simulink model "proba1"  (Simulink 7.0)
settings: Solver=ode1  StartTime=0.0  StopTime=Inf  FixedStep=0.001  RelTol=1e-3
PostLoadFcn:
  | ,try, rti_mdl_postloadfcn(bdroot, 'UpdateModel', 280, 'rti1005'); catch, disp(lasterr); end,
libraries: simulink x27, simulink_extras x12, rtilibm x10
(part 1 of 2)
settings Model: Creator=k12_p800a  LastModifiedBy=k12_p800a  BufferReuse=off
settings OptimizationCC: BlockReduction=off  BooleanDataType=off  OptimizeBlockIOStorage=off  BufferReuse=off  ExpressionFolding=off  LocalBlockOutputs=off
settings HardwareCC: ProdIntDivRoundTo=Zero  ProdEndianess=BigEndian  ProdHWDeviceType=Specified  TargetIntDivRoundTo=Zero  TargetEndianess=BigEndian
settings RTWCC: SystemTargetFile=rti1005.tlc  MakeCommand=make_rti  TemplateMakefile=rti1005.tmf  Description=dSPACE DS1005 Hardware Platform  ProcessScript=rti1005_make_rtw_hook
settings STFCustomTargetCC: GenFloatMathFcnCalls=ANSI_C  ModelReferenceCompliant=off  SystemTargetFile=rti1005.tlc
settings GRTTargetCC: ModelReferenceCompliant=off  CompOptLevelCompliant=off  MatFileLogging=off  ExtModeMexFile=rti_comm_2
settings CustomProperty: DataType=RTWOptions_EnumType_C__dSPACE_60_matlab_rti1005_tlc_rti1005_InitialSimState  Value=RUN
settings EnumStrPairs: String=RUN

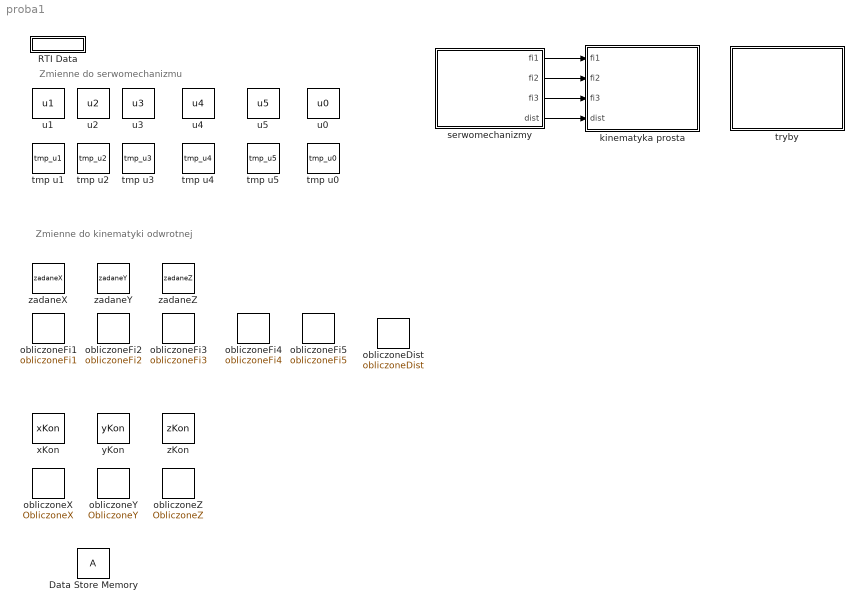
== system proba1 ==
  note: Zmienne do kinematyki odwrotnej
  note: Zmienne do serwomechanizmu
  Data Store Memory : DataStoreMemory  DataStoreName=A  ReadBeforeWriteMsg=warning  WriteAfterWriteMsg=warning  WriteAfterReadMsg=warning  OutDataType=sfix(16)  OutScaling=2^0
  RTI Data : Subsystem  Tag=struct('RTIDataServer',struct('RTIDataServerVs','2','RTIModelDescription','struct(''main'',''proba1'',''sub'','''',''isMp'',0)'))  LoadFcn="if exist('rtidc'), try,  rtidc('DataHostBlockClbLoad', gcbh); catch, disp(['Warning: ''LoadFcn'' for RTI Data block failed: ' lasterr]); end, end,"
      settings: CopyFcn="if exist('rtidc'), try,  rtidc('DataHostBlockClbCopy', gcbh); catch, disp(['Warning: ''CopyFcn'' for RTI Data block failed: ' lasterr]); end, end,"  DeleteFcn="if exist('rtidc'), try,  rtidc('DataHostBlockClbDelete', gcbh); catch, disp(['Warning: ''DeleteFcn'' for RTI Data block failed: ' lasterr]); end, end,"  ModelCloseFcn="if exist('rtidc'), try,  rtidc('DataHostBlockClbModelClose', gcbh); catch, disp(['Warning: ''ModelCloseFcn'' for RTI Data block failed: ' lasterr]); end, end,"  PreSaveFcn="if exist('rtidc'), try,  rtidc('DataHostBlockClbPreSave', gcbh); catch, disp(['Warning: ''PreSaveFcn'' for RTI Data block failed: ' lasterr]); end, end,"  PostSaveFcn="if exist('rtidc'), try,  rtidc('DataHostBlockClbPostSave', gcbh); catch, disp(['Warning: ''PostSaveFcn'' for RTI Data block failed: ' lasterr]); end, end,"  NameChangeFcn="if exist('rtidc'), try,  rtidc('DataHostBlockClbNameChange', gcbh); catch, disp(['Warning: ''NameChangeFcn'' for RTI Data block failed: ' lasterr]); end, end,"
      mask Type: RTI_DATA_HOST
      mask Description:
      | RTI Data Block.
      | This block is used by RTI to store internal model-dependent data.
      | Please keep this block on the root level of the model. Deleting this block will result in data loss.
      | 
      | NEVER DELETE OR COPY THIS BLOCK!
      mask Help:
      | RTI Data Block.
      | This block is used by RTI to store internal model-dependent data.
      | Please keep this block on the root level of the model. Deleting this block will result in data loss.
      | 
      | NEVER DELETE OR COPY THIS BLOCK!
      mask Display:
      | text(0.5, 0.5, 'RTI Data', 'HorizontalAlignment', 'center');
      | plot([1 0]);
  kinematyka prosta : Subsystem
  obliczoneDist : DataStoreMemory  DataStoreName=obliczoneDist  ReadBeforeWriteMsg=warning  WriteAfterWriteMsg=warning  WriteAfterReadMsg=warning
  obliczoneFi1 : DataStoreMemory  DataStoreName=obliczoneFi1  ReadBeforeWriteMsg=warning  WriteAfterWriteMsg=warning  WriteAfterReadMsg=warning
  obliczoneFi2 : DataStoreMemory  DataStoreName=obliczoneFi2  ReadBeforeWriteMsg=warning  WriteAfterWriteMsg=warning  WriteAfterReadMsg=warning
  obliczoneFi3 : DataStoreMemory  DataStoreName=obliczoneFi3  ReadBeforeWriteMsg=warning  WriteAfterWriteMsg=warning  WriteAfterReadMsg=warning
  obliczoneFi4 : DataStoreMemory  DataStoreName=obliczoneFi4  ReadBeforeWriteMsg=warning  WriteAfterWriteMsg=warning  WriteAfterReadMsg=warning
  obliczoneFi5 : DataStoreMemory  DataStoreName=obliczoneFi5  ReadBeforeWriteMsg=warning  WriteAfterWriteMsg=warning  WriteAfterReadMsg=warning
  obliczoneX : DataStoreMemory  DataStoreName=ObliczoneX  ReadBeforeWriteMsg=warning  WriteAfterWriteMsg=warning  WriteAfterReadMsg=warning
  obliczoneY : DataStoreMemory  DataStoreName=ObliczoneY  ReadBeforeWriteMsg=warning  WriteAfterWriteMsg=warning  WriteAfterReadMsg=warning
  obliczoneZ : DataStoreMemory  DataStoreName=ObliczoneZ  ReadBeforeWriteMsg=warning  WriteAfterWriteMsg=warning  WriteAfterReadMsg=warning
  serwomechanizmy : Subsystem
  tmp u0 : DataStoreMemory  DataStoreName=tmp_u0  ReadBeforeWriteMsg=warning  WriteAfterWriteMsg=warning  WriteAfterReadMsg=warning
  tmp u1 : DataStoreMemory  DataStoreName=tmp_u1  ReadBeforeWriteMsg=warning  WriteAfterWriteMsg=warning  WriteAfterReadMsg=warning
  tmp u2 : DataStoreMemory  DataStoreName=tmp_u2  ReadBeforeWriteMsg=warning  WriteAfterWriteMsg=warning  WriteAfterReadMsg=warning
  tmp u3 : DataStoreMemory  DataStoreName=tmp_u3  ReadBeforeWriteMsg=warning  WriteAfterWriteMsg=warning  WriteAfterReadMsg=warning
  tmp u4 : DataStoreMemory  DataStoreName=tmp_u4  ReadBeforeWriteMsg=warning  WriteAfterWriteMsg=warning  WriteAfterReadMsg=warning
  tmp u5 : DataStoreMemory  DataStoreName=tmp_u5  ReadBeforeWriteMsg=warning  WriteAfterWriteMsg=warning  WriteAfterReadMsg=warning
  tryby : Subsystem
  u0 : DataStoreMemory  DataStoreName=u0  ReadBeforeWriteMsg=warning  WriteAfterWriteMsg=warning  WriteAfterReadMsg=warning
  u1 : DataStoreMemory  DataStoreName=u1  ReadBeforeWriteMsg=warning  WriteAfterWriteMsg=warning  WriteAfterReadMsg=warning
  u2 : DataStoreMemory  DataStoreName=u2  ReadBeforeWriteMsg=warning  WriteAfterWriteMsg=warning  WriteAfterReadMsg=warning
  u3 : DataStoreMemory  DataStoreName=u3  ReadBeforeWriteMsg=warning  WriteAfterWriteMsg=warning  WriteAfterReadMsg=warning
  u4 : DataStoreMemory  DataStoreName=u4  ReadBeforeWriteMsg=warning  WriteAfterWriteMsg=warning  WriteAfterReadMsg=warning
  u5 : DataStoreMemory  DataStoreName=u5  ReadBeforeWriteMsg=warning  WriteAfterWriteMsg=warning  WriteAfterReadMsg=warning
  xKon : DataStoreMemory  DataStoreName=xKon  ReadBeforeWriteMsg=warning  WriteAfterWriteMsg=warning  WriteAfterReadMsg=warning
  yKon : DataStoreMemory  DataStoreName=yKon  ReadBeforeWriteMsg=warning  WriteAfterWriteMsg=warning  WriteAfterReadMsg=warning
  zKon : DataStoreMemory  DataStoreName=zKon  ReadBeforeWriteMsg=warning  WriteAfterWriteMsg=warning  WriteAfterReadMsg=warning
  zadaneX : DataStoreMemory  DataStoreName=zadaneX  ReadBeforeWriteMsg=warning  WriteAfterWriteMsg=warning  WriteAfterReadMsg=warning
  zadaneY : DataStoreMemory  DataStoreName=zadaneY  ReadBeforeWriteMsg=warning  WriteAfterWriteMsg=warning  WriteAfterReadMsg=warning
  zadaneZ : DataStoreMemory  DataStoreName=zadaneZ  ReadBeforeWriteMsg=warning  WriteAfterWriteMsg=warning  WriteAfterReadMsg=warning
  wires:
  serwomechanizmy/1(fi1) -> kinematyka prosta/1(fi1)
  serwomechanizmy/2(fi2) -> kinematyka prosta/2(fi2)
  serwomechanizmy/3(fi3) -> kinematyka prosta/3(fi3)
  serwomechanizmy/4(dist) -> kinematyka prosta/4(dist)

== system proba1/RTI Data ==
  RTI Data Store : Subsystem  Tag="struct('private',struct('version',struct('dsVer',uint32(2),'dsVerCreation',uint32(2),'RTI',struct('ver','5.6','type','RTI1005')),'access',struct('type','Model','isPerm',1,'created',['12-Mar-2012 08:50:59'],'modified',['07-May-2014 13:55:27'],'location','')),'public',struct('main',struct('data',[]),'sub',struct('name',{{'proba1'}},'data',{{struct('TH',struct('thTaskInfo',struct('taskType',{'TIMER','HWINT','TMRINT','SWINT'},'tasksNumOf',{1,0,0,0},'srcIds',{{'TIMERA'},{},{},{}},'taskNames',{{['Timer Task 1']},{},{},{}})),'th_tc',struct('dataType','TASK','taskGroupId','','taskGroupList',{{}},'taskSchedulingPolicy','FCFS','taskType','TIMER','blkh',-1,'srcId','TIMERA','srcSgnName',['Timer A interrupt'],'srcCpuName','','taskName',['Timer Task 1  [0.001] s'],'taskNameDisplayExt','','smplTime',0.001,'smplTimeOffs',0,'hasFixedPriority',0,'priority',1,'hasFixedOvc',0,'ovcType',1,'ovcMax',1),'tc_th',struct('dataType','TASK','taskGroupId','','taskGroupList',{{}},'taskSchedulingPolicy','FCFS','taskType','TIMER','blkh',-1,'srcId','TIMERA','srcSgnName',['Timer A interrupt'],'srcCpuName','','taskName',['Timer Task 1  [0.001] s'],'taskNameDisplayExt','','smplTime',0.001,'smplTimeOffs',0,'hasFixedPriority',0,'priority',1,'hasFixedOvc',0,'ovcType',1,'ovcMax',1),'VersionInfo',struct('verStr',['-------------------------------------------------------------------------------------' char(10) 'MATLAB Version 7.5.0.342 (R2007b)' char(10) 'Operating System: Microsoft Windows 2000 Version 5.0 (Build 2195: Service Pack 4)' char(10) 'Java VM Version: Java 1.6.0 with Sun Microsystems Inc. Java HotSpot(TM) Client VM mixed mode' char(10) '-------------------------------------------------------------------------------------' char(10) 'MATLAB' blanks(48) 'Version 7.5        (R2007b)' char(10) 'Simulink' blanks(46) 'Version 7.0        (R2007b)' char(10) 'Communications Blockset' blanks(31) 'Version 3.6        (R2007b)' char(10) 'Communications Toolbox' blanks(32) 'Version 4.0        (R2007b)' char(10) 'Control System Toolbox' blanks(32) 'Version 8.0.1      (R2007b)' char(10) 'Curve Fitting Toolbox' blanks(33) 'Version 1.2        (R2007b)' char(10) 'Data Acquisition Toolbox' blanks(30) 'Version 2.11       (R2007b)' char(10) 'Extended Symbolic Math Toolbox' blanks(24) 'Version 3.2.2      (R2007b)' char(10) 'Filter Design Toolbox' blanks(33) 'Version 4.2        (R2007b)' char(10) 'Financial Derivatives Toolbox' blanks(25) 'Version 5.1        (R2007b)' char(10) 'Financial Toolbox' blanks(37) 'Version 3.3        (R2007b)' char(10) 'Fixed-Point Toolbox' blanks(35) 'Version 2.1        (R2007b)' char(10) 'Fuzzy Logic Toolbox' blanks(35) 'Version 2.2.6      (R2007b)' char(10) 'Gauges Blockset' blanks(39) 'Version 2.0.5      (R2007b)' char(10) 'Image Acquisition Toolbox' blanks(29) 'Version 3.0        (R2007b)' char(10) 'Image Processing Toolbox' blanks(30) 'Version 6.0        (R2007b)' char(10) 'Instrument Control Toolbox' blanks(28) 'Version 2.5        (R2007b)' char(10) 'Link for Code Composer Studio' blanks(25) 'Version 3.1        (R2007b)' char(10) 'MATLAB Builder for .NET' blanks(31) 'Version 2.2.1      (R2007b)' char(10) 'MATLAB Compiler' blanks(39) 'Version 4.7        (R2007b)' char(10) 'Model Predictive Control Toolbox' blanks(22) 'Version 2.3        (R2007b)' char(10) 'Neural Network Toolbox' blanks(32) 'Version 5.1        (R2007b)' char(10) 'Optimization Toolbox' blanks(34) 'Version 3.1.2      (R2007b)' char(10) 'Partial Differential Equation Toolbox' blanks(17) 'Version 1.0.11     (R2007b)' char(10) 'Real-Time Windows Target' blanks(30) 'Version 3.0        (R2007b)' char(10) 'Real-Time Workshop' blanks(36) 'Version 7.0        (R2007b)' char(10) 'Robust Control Toolbox' blanks(32) 'Version 3.3        (R2007b)' char(10) 'Signal Processing Blockset' blanks(28) 'Version 6.6        (R2007b)' char(10) 'Signal Processing Toolbox' blanks(29) 'Version 6.8        (R2007b)' char(10) 'SimMechanics' blanks(42) 'Version 2.7        (R2007b)' char(10) 'SimPowerSystems' blanks(39) 'Version 4.5        (R2007b)' char(10) 'Simscape' blanks(46) 'Version 2.0        (R2007b)' char(10) 'Simulink Control Design' blanks(31) 'Version 2.2        (R2007b)' char(10) 'Simulink Fixed Point' blanks(34) 'Version 5.5        (R2007b)' char(10) 'Simulink Response Optimization' blanks(24) 'Version 3.1.2      (R2007b)' char(10) 'Spline Toolbox' blanks(40) 'Version 3.3.3      (R2007b)' char(10) 'Stateflow' blanks(45) 'Version 7.0        (R2007b)' char(10) 'Stateflow Coder' blanks(39) 'Version 7.0        (R2007b)' char(10) 'Statistics Toolbox' blanks(36) 'Version 6.1        (R2007b)' char(10) 'Symbolic Math Toolbox' blanks(33) 'Version 3.2.2      (R2007b)' char(10) 'System Identification Toolbox' blanks(25) 'Version 7.1        (R2007b)' char(10) 'Target for TI C6000(tm)' blanks(31) 'Version 3.3        (R2007b)' char(10) 'Video and Image Processing Blockset' blanks(19) 'Version 2.4        (R2007b)' char(10) 'Wavelet Toolbox' blanks(39) 'Version 4.1        (R2007b)' char(10) 'dSPACE ControlDesk to Simulink Interface' blanks(14) 'Version 3.2' blanks(16) '' char(10) 'dSPACE MLIB/MTRACE MATLAB-dSPACE Interface Libr...    Version 4.6.4' blanks(14) '' char(10) 'dSPACE MotionDesk Blockset' blanks(28) 'Version 1.3.9' blanks(14) '' char(10) 'dSPACE Real-Time Interface (RTI1005)' blanks(18) 'Version 5.6' blanks(16) '' char(10) '' char(10) 'Trademarks' char(10) '------------------' char(10) 'MATLAB, Simulink, Stateflow, Handle Graphics, Real-Time Workshop, and xPC' char(10) 'TargetBox are registered trademarks and SimBiology, SimEvents, and' char(10) 'SimHydraulics are trademarks of The MathWorks, Inc. Other product or' char(10) 'brand names are trademarks or registered trademarks of their respective' char(10) 'holders. ' char(10) ''],'mlVerStr',['7.5.0.342 (R2007b)'],'rtiVerStr',['RTI1005 5.6 (16-Nov-2007)'],'rtiMdlVer',280))}})))"
      mask Type: RTI_DATA_STORE
      mask Description:
      | RTI Data Store Block. This block is used by RTI to store internal model dependent data. Deleting this block will result in data loss.
      | 
      | NEVER DELETE, COPY, OR MODIFY THIS BLOCK!
      mask Help:
      | RTI Data Store Block. This block is used by RTI to store internal model dependent data. Deleting this block will result in data loss.
      | 
      | NEVER DELETE, COPY, OR MODIFY THIS BLOCK!
      mask Display: text(0.5, 0.5, ' ', 'HorizontalAlignment', 'center');

== system proba1/kinematyka prosta ==
  fi1 : Inport
  fi2 : Inport  Port=2
  fi3 : Inport  Port=3
  dist : Inport  Port=4
  Data Store Write : DataStoreWrite  DataStoreName=xKon  SampleTime=-1
  Data Store Write1 : DataStoreWrite  DataStoreName=yKon  SampleTime=-1
  Data Store Write2 : DataStoreWrite  DataStoreName=zKon  SampleTime=-1
  Degrees to Radians : simulink_extras/Transformations/Degrees to Radians  SystemSampleTime=-1
  Degrees to Radians1 : simulink_extras/Transformations/Degrees to Radians  SystemSampleTime=-1
  Degrees to Radians2 : simulink_extras/Transformations/Degrees to Radians  SystemSampleTime=-1
  Mux : Mux  Inputs=3
  Sum : Sum  Inputs=++|  OutDataType=sfix(16)  OutScaling=2^0
  x : Fcn  Expr=cos(u(1))*(670*cos(-u(3)) + 450*cos(3.14159/2 - u(2)))
  y : Fcn  Expr=sin(u(1))*(670*cos(-u(3)) + 450*cos(3.14159/2 - u(2)))
  z : Fcn  Expr=670*sin(-u(3)) + 450*sin(3.14159/2 - u(2)) + 700
  wires:
  fi1/1 -> Degrees to Radians/1
  Degrees to Radians1/1 -> Mux/2
  fi2/1 -> Degrees to Radians1/1
  fi3/1 -> Degrees to Radians2/1
  Degrees to Radians/1 -> Mux/1
  Degrees to Radians2/1 -> Mux/3
  z/1 -> Data Store Write2/1
  x/1 -> Data Store Write/1
  Mux/1 -> y/1, x/1, z/1
  Sum/1 -> Data Store Write1/1
  dist/1 -> Sum/1
  y/1 -> Sum/2

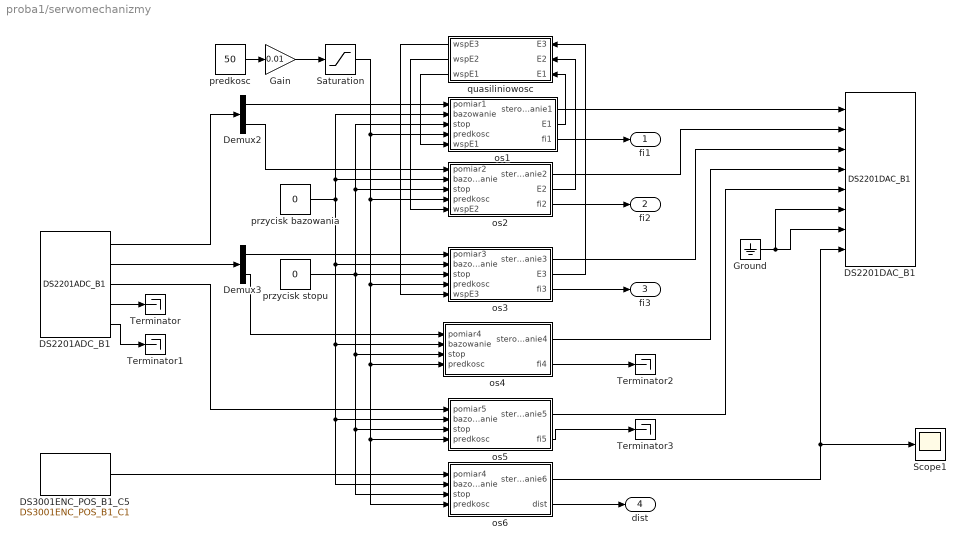
== system proba1/serwomechanizmy ==
  DS2201ADC_B1 : rtilibm/DS2201/DS2201ADC_B1  SystemSampleTime=-1  BoardNo=1  channelNo1=[1 2 3 4]  channelNo2=[5 6 7 8]  channelNo3=[9 10]  channelNo4=-1  channelNo5=-1  DialogFcn=gui2201adc  UnitName={'DS2201ADC_B'}  UnitValues={ 1 }  DSProperties=struct('RTI',struct('Version',uint32(1),'BlockType',struct('isSLSource',uint8(1),'isSLSink',uint8(0),'isHWSource',uint8(1),'isHWSink',uint8(0),'isSetup',uint8(0),'isInline',uint8(1),'isNonInline',uint8(0),'isInterrupt',uint8(0),'isChannelwise',uint8(0)),'IOBoardType','DS2201','UnitType','ADC','Identifier','ADCMUX','DialogType','ML','BlockSet','NONE','SlaveProcessor','NONE'))
  DS2201DAC_B1 : rtilibm/DS2201/DS2201DAC_B1  SystemSampleTime=-1  BoardNo=1  IOErrorMode=[0 0]  InitValue=[0 0 0 0 0 0 0 0]  TermMode=[0 0 0 0 0 0 0 0]  TermValue=[0 0 0 0 0 0 0 0]  DialogFcn=gui2201dac  UnitName={'DS2201DAC_B'}  UnitValues={ 1 }  DSProperties=struct('RTI',struct('Version',uint32(1),'BlockType',struct('isSLSource',uint8(0),'isSLSink',uint8(1),'isHWSource',uint8(0),'isHWSink',uint8(1),'isSetup',uint8(0),'isInline',uint8(1),'isNonInline',uint8(0),'isInterrupt',uint8(0),'isChannelwise',uint8(0)),'IOBoardType','DS2201','UnitType','DAC','Identifier','DAC','DialogType','ML','BlockSet','NONE','SlaveProcessor','NONE'))
  DS3001ENC_POS_B1_C5 : rtilibm/DS3001/DS3001ENC_POS_B1_C1  SystemSampleTime=-1  BoardNo=1  ChannelNo=5  DialogFcn=gui3001enc_xpos_c  UnitName={ 'DS3001ENC_POS_B' , '_C'}  UnitValues="{ 1  5 }"  DSProperties=struct('RTI',struct('Version',uint32(1),'BlockType',struct('isSLSource',uint8(1),'isSLSink',uint8(0),'isHWSource',uint8(1),'isHWSink',uint8(0),'isSetup',uint8(0),'isInline',uint8(1),'isNonInline',uint8(0),'isInterrupt',uint8(0),'isChannelwise',uint8(1)),'IOBoardType','DS3001','UnitType','ENC','Identifier','ENCPOSCH','DialogType','ML','BlockSet','NONE','SlaveProcessor','NONE'))
      settings: SignalType=1
  Demux2 : Demux  Outputs=2
  Demux3 : Demux  Outputs=2
  Gain : Gain  Gain=0.01
  Ground : Ground
  Saturation : Saturate  UpperLimit=1  LowerLimit=0.01
  Scope1 : Scope
  Terminator{,1..3} (4 alike) : Terminator
  os1 : Subsystem
  os2 : Subsystem
  os3 : Subsystem
  os4 : Subsystem
  os5 : Subsystem
  os6 : Subsystem
  predkosc : Constant  Value=50
  przycisk bazowania : Constant  Value=0
  przycisk stopu : Constant  Value=0
  quasiliniowosc : Subsystem  Orientation=left
  fi1 : Outport
  fi2 : Outport  Port=2
  fi3 : Outport  Port=3
  dist : Outport  Port=4
  wires:
  DS2201ADC_B1/1 -> Demux2/1
  DS2201ADC_B1/2 -> Demux3/1
  Demux3/1 -> os3/1(pomiar3)
  DS2201ADC_B1/3 -> os5/1(pomiar5)
  Demux2/1 -> os1/1(pomiar1)
  Demux3/2 -> os4/1(pomiar4)
  DS2201ADC_B1/4 -> Terminator/1
  DS2201ADC_B1/5 -> Terminator1/1
  Ground/1 -> DS2201DAC_B1/7, DS2201DAC_B1/6
  Gain/1 -> Saturation/1
  os1/1(sterowanie1) -> DS2201DAC_B1/1
  os2/1(sterowanie2) -> DS2201DAC_B1/2
  os3/1(sterowanie3) -> DS2201DAC_B1/3
  os4/1(sterowanie4) -> DS2201DAC_B1/4
  Saturation/1 -> os1/4(predkosc), os2/4(predkosc), os3/4(predkosc), os4/4(predkosc), os6/4(predkosc), os5/4(predkosc)
  przycisk stopu/1 -> os2/3(stop), os1/3(stop), os3/3(stop), os4/3(stop), os6/3(stop), os5/3(stop)
  Demux2/2 -> os2/1(pomiar2)
  przycisk bazowania/1 -> os1/2(bazowanie), os2/2(bazowanie), os3/2(bazowanie), os4/2(bazowanie), os6/2(bazowanie), os5/2(bazowanie)
  predkosc/1 -> Gain/1
  os2/3(fi2) -> fi2/1
  os3/3(fi3) -> fi3/1
  os1/3(fi1) -> fi1/1
  DS3001ENC_POS_B1_C5/1 -> os6/1(pomiar4)
  os6/1(sterowanie6) -> DS2201DAC_B1/8, Scope1/1
  quasiliniowosc/3(wspE1) -> os1/5(wspE1)
  quasiliniowosc/2(wspE2) -> os2/5(wspE2)
  quasiliniowosc/1(wspE3) -> os3/5(wspE3)
  os6/2(dist) -> dist/1
  os1/2(E1) -> quasiliniowosc/3(E1)
  os2/2(E2) -> quasiliniowosc/2(E2)
  os3/2(E3) -> quasiliniowosc/1(E3)
  os4/2(fi4) -> Terminator2/1
  os5/1(sterowanie5) -> DS2201DAC_B1/5
  os5/2(fi5) -> Terminator3/1

== system proba1/tryby ==
  Compare To Constant : simulink/Logic and Bit Operations/Compare To Constant  SystemSampleTime=-1  relop===  const=0  LogicOutDataTypeMode=uint8
  Compare To Constant1 : simulink/Logic and Bit Operations/Compare To Constant  SystemSampleTime=-1  relop===  const=1  LogicOutDataTypeMode=uint8
  Compare To Constant2 : simulink/Logic and Bit Operations/Compare To Constant  SystemSampleTime=-1  relop===  const=2  LogicOutDataTypeMode=uint8
  Compare To Constant3 : simulink/Logic and Bit Operations/Compare To Constant  SystemSampleTime=-1  relop===  const=3  LogicOutDataTypeMode=uint8
  Logical Operator : Logic  Orientation=down  Operator=OR  AllPortsSameDT=off  OutDataTypeMode=boolean
  jedz do przedmiotu : Subsystem  TreatAsAtomicUnit=on
  kinematyka odwrotna : Subsystem  TreatAsAtomicUnit=on
  przycisk jedz do przedmiotu : Constant  Value=0
  przycisk rozpoznawanie obrazu : Constant  Value=0
  przycisk wyzwolenia : Constant  Value=0
  rozpoznawanie obrazu : Subsystem  TreatAsAtomicUnit=on
  tryb ciagly : Subsystem  TreatAsAtomicUnit=on
  tryb kinematyki odwrotnej : Subsystem  TreatAsAtomicUnit=on
  tryb wyzwalany : Subsystem  TreatAsAtomicUnit=on
  wybor trybu : Constant  Value=0
  wires:
  Compare To Constant/1 -> tryb ciagly/Enable
  Compare To Constant1/1 -> tryb wyzwalany/Enable
  wybor trybu/1 -> Compare To Constant/1, Compare To Constant1/1, Compare To Constant2/1, Compare To Constant3/1
  przycisk wyzwolenia/1 -> tryb wyzwalany/Trigger, tryb kinematyki odwrotnej/Trigger
  Compare To Constant2/1 -> tryb kinematyki odwrotnej/Enable, Logical Operator/1, kinematyka odwrotna/1(In1)
  Compare To Constant3/1 -> rozpoznawanie obrazu/Enable, jedz do przedmiotu/Enable
  przycisk rozpoznawanie obrazu/1 -> rozpoznawanie obrazu/Trigger
  przycisk jedz do przedmiotu/1 -> jedz do przedmiotu/Trigger
  rozpoznawanie obrazu/1(gotowy) -> Logical Operator/2
  Logical Operator/1 -> kinematyka odwrotna/Enable

== system proba1/RTI Data/RTI Data Store ==
  RTI Data Store : Subsystem
      mask Type: RTI_DATA_STORE
      mask Description:
      | RTI Data Store Block. This block is used by RTI to store internal model dependent data. Deleting this block will result in data loss.
      | 
      | NEVER DELETE, COPY, OR MODIFY THIS BLOCK!
      mask Help:
      | RTI Data Store Block. This block is used by RTI to store internal model dependent data. Deleting this block will result in data loss.
      | 
      | NEVER DELETE, COPY, OR MODIFY THIS BLOCK!
      mask Display: text(0.5, 0.5, ' ', 'HorizontalAlignment', 'center');

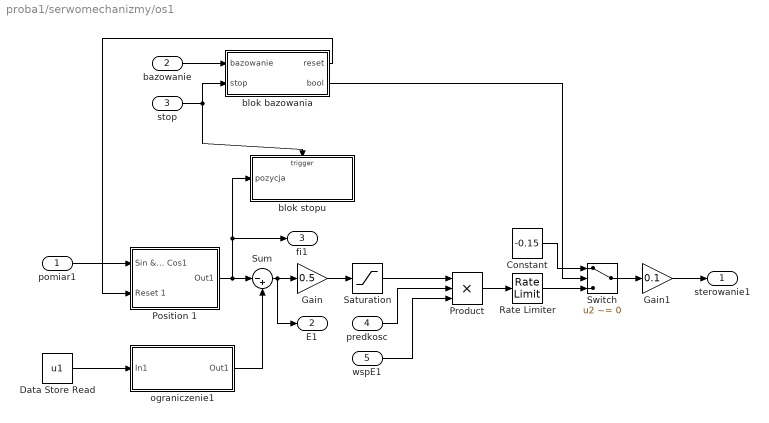
== system proba1/serwomechanizmy/os1 ==
  pomiar1 : Inport
  bazowanie : Inport  Port=2
  stop : Inport  Port=3
  predkosc : Inport  Port=4
  wspE1 : Inport  Port=5
  Constant : Constant  Value=-0.15
  Data Store Read : DataStoreRead  DataStoreName=u1  SampleTime=0
  Gain : Gain  Gain=0.5
  Gain1 : Gain  Gain=0.1
  Position 1 : Subsystem
  Product : Product  Inputs=3  RndMeth=Zero
  Rate Limiter : RateLimiter  RisingSlewLimit=50  FallingSlewLimit=-50  SampleTimeMode=inherited
  Saturation : Saturate  UpperLimit=3  LowerLimit=-3
  Sum : Sum  Inputs=|-+
  Switch : Switch  Criteria=u2 ~= 0
  blok bazowania : Subsystem
  blok stopu : Subsystem  TreatAsAtomicUnit=on
  ograniczenie1 : Subsystem
  sterowanie1 : Outport
  E1 : Outport  Port=2
  fi1 : Outport  Port=3
  wires:
  Sum/1 -> Gain/1, E1/1
  pomiar1/1 -> Position 1/1(Sin && Cos1)
  Position 1/1(Out1) -> Sum/1, blok stopu/1(pozycja), fi1/1
  Gain1/1 -> sterowanie1/1
  Data Store Read/1 -> ograniczenie1/1(In1)
  ograniczenie1/1(Out1) -> Sum/2
  Gain/1 -> Saturation/1
  Saturation/1 -> Product/1
  predkosc/1 -> Product/2
  wspE1/1 -> Product/3
  Product/1 -> Rate Limiter/1
  Constant/1 -> Switch/1
  Switch/1 -> Gain1/1
  Rate Limiter/1 -> Switch/3
  blok bazowania/2(bool) -> Switch/2
  blok bazowania/1(reset) -> Position 1/2(Reset 1)
  bazowanie/1 -> blok bazowania/1(bazowanie)
  stop/1 -> blok bazowania/2(stop), blok stopu/Trigger

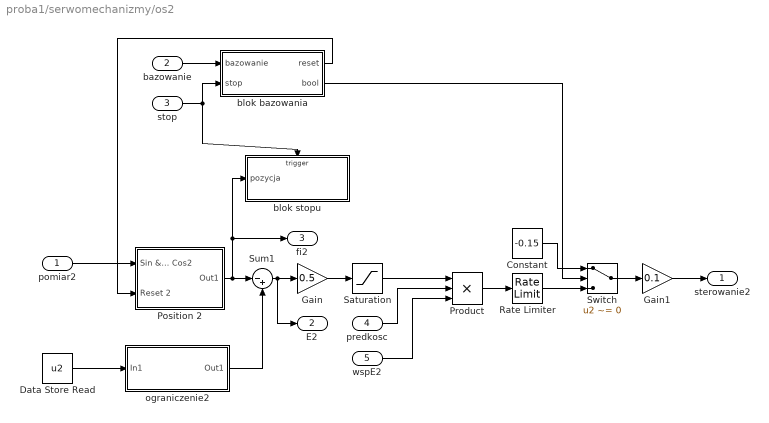
== system proba1/serwomechanizmy/os2 ==
  pomiar2 : Inport
  bazowanie : Inport  Port=2
  stop : Inport  Port=3
  predkosc : Inport  Port=4
  wspE2 : Inport  Port=5
  Constant : Constant  Value=-0.15
  Data Store Read : DataStoreRead  DataStoreName=u2  SampleTime=0
  Gain : Gain  Gain=0.5
  Gain1 : Gain  Gain=0.1
  Position 2 : Subsystem
  Product : Product  Inputs=3  RndMeth=Zero
  Rate Limiter : RateLimiter  RisingSlewLimit=50  FallingSlewLimit=-50  SampleTimeMode=inherited
  Saturation : Saturate  UpperLimit=3  LowerLimit=-3
  Sum1 : Sum  Inputs=|-+
  Switch : Switch  Criteria=u2 ~= 0
  blok bazowania : Subsystem
  blok stopu : Subsystem  TreatAsAtomicUnit=on
  ograniczenie2 : Subsystem
  sterowanie2 : Outport
  E2 : Outport  Port=2
  fi2 : Outport  Port=3
  wires:
  Sum1/1 -> Gain/1, E2/1
  pomiar2/1 -> Position 2/1(Sin && Cos2)
  Position 2/1(Out1) -> Sum1/1, fi2/1, blok stopu/1(pozycja)
  Gain1/1 -> sterowanie2/1
  Data Store Read/1 -> ograniczenie2/1(In1)
  ograniczenie2/1(Out1) -> Sum1/2
  Gain/1 -> Saturation/1
  Saturation/1 -> Product/1
  predkosc/1 -> Product/2
  wspE2/1 -> Product/3
  Product/1 -> Rate Limiter/1
  Constant/1 -> Switch/1
  Switch/1 -> Gain1/1
  Rate Limiter/1 -> Switch/3
  blok bazowania/2(bool) -> Switch/2
  blok bazowania/1(reset) -> Position 2/2(Reset 2)
  bazowanie/1 -> blok bazowania/1(bazowanie)
  stop/1 -> blok stopu/Trigger, blok bazowania/2(stop)

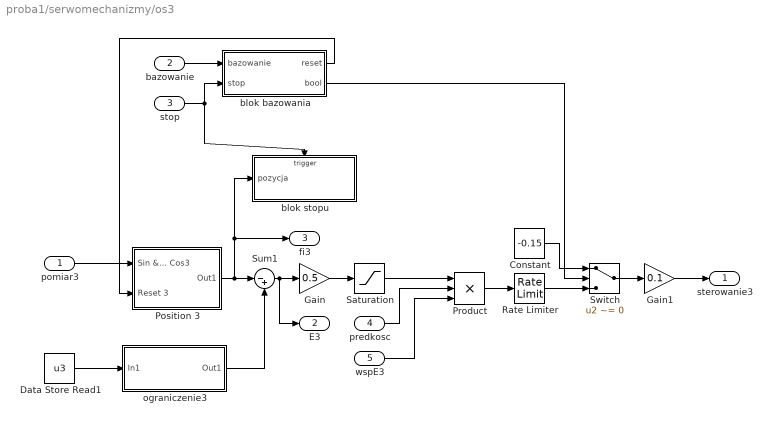
== system proba1/serwomechanizmy/os3 ==
  pomiar3 : Inport
  bazowanie : Inport  Port=2
  stop : Inport  Port=3
  predkosc : Inport  Port=4
  wspE3 : Inport  Port=5
  Constant : Constant  Value=-0.15
  Data Store Read1 : DataStoreRead  DataStoreName=u3  SampleTime=0
  Gain : Gain  Gain=0.5
  Gain1 : Gain  Gain=0.1
  Position 3 : Subsystem
  Product : Product  Inputs=3  RndMeth=Zero
  Rate Limiter : RateLimiter  RisingSlewLimit=50  FallingSlewLimit=-50  SampleTimeMode=inherited
  Saturation : Saturate  UpperLimit=3  LowerLimit=-3
  Sum1 : Sum  Inputs=|-+
  Switch : Switch  Criteria=u2 ~= 0
  blok bazowania : Subsystem
  blok stopu : Subsystem  TreatAsAtomicUnit=on
  ograniczenie3 : Subsystem
  sterowanie3 : Outport
  E3 : Outport  Port=2
  fi3 : Outport  Port=3
  wires:
  Sum1/1 -> Gain/1, E3/1
  pomiar3/1 -> Position 3/1(Sin && Cos3)
  Position 3/1(Out1) -> Sum1/1, fi3/1, blok stopu/1(pozycja)
  Gain1/1 -> sterowanie3/1
  Data Store Read1/1 -> ograniczenie3/1(In1)
  ograniczenie3/1(Out1) -> Sum1/2
  Gain/1 -> Saturation/1
  Saturation/1 -> Product/1
  predkosc/1 -> Product/2
  wspE3/1 -> Product/3
  Product/1 -> Rate Limiter/1
  Constant/1 -> Switch/1
  Switch/1 -> Gain1/1
  Rate Limiter/1 -> Switch/3
  blok bazowania/2(bool) -> Switch/2
  blok bazowania/1(reset) -> Position 3/2(Reset 3)
  bazowanie/1 -> blok bazowania/1(bazowanie)
  stop/1 -> blok stopu/Trigger, blok bazowania/2(stop)

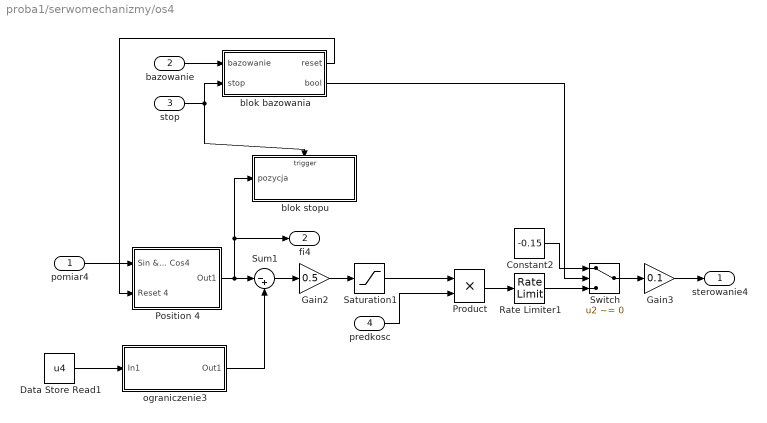
== system proba1/serwomechanizmy/os4 ==
  pomiar4 : Inport
  bazowanie : Inport  Port=2
  stop : Inport  Port=3
  predkosc : Inport  Port=4
  Constant2 : Constant  Value=-0.15
  Data Store Read1 : DataStoreRead  DataStoreName=u4  SampleTime=0
  Gain2 : Gain  Gain=0.5
  Gain3 : Gain  Gain=0.1
  Position 4 : Subsystem
  Product : Product  RndMeth=Zero
  Rate Limiter1 : RateLimiter  RisingSlewLimit=50  FallingSlewLimit=-50  SampleTimeMode=inherited
  Saturation1 : Saturate  UpperLimit=3  LowerLimit=-3
  Sum1 : Sum  Inputs=|-+
  Switch : Switch  Criteria=u2 ~= 0
  blok bazowania : Subsystem
  blok stopu : Subsystem  TreatAsAtomicUnit=on
  ograniczenie3 : Subsystem
  sterowanie4 : Outport
  fi4 : Outport  Port=2
  wires:
  Sum1/1 -> Gain2/1
  pomiar4/1 -> Position 4/1(Sin && Cos4)
  Position 4/1(Out1) -> Sum1/1, fi4/1, blok stopu/1(pozycja)
  Gain3/1 -> sterowanie4/1
  Data Store Read1/1 -> ograniczenie3/1(In1)
  ograniczenie3/1(Out1) -> Sum1/2
  Gain2/1 -> Saturation1/1
  Saturation1/1 -> Product/1
  predkosc/1 -> Product/2
  Product/1 -> Rate Limiter1/1
  Constant2/1 -> Switch/1
  Switch/1 -> Gain3/1
  Rate Limiter1/1 -> Switch/3
  blok bazowania/2(bool) -> Switch/2
  blok bazowania/1(reset) -> Position 4/2(Reset 4)
  bazowanie/1 -> blok bazowania/1(bazowanie)
  stop/1 -> blok stopu/Trigger, blok bazowania/2(stop)

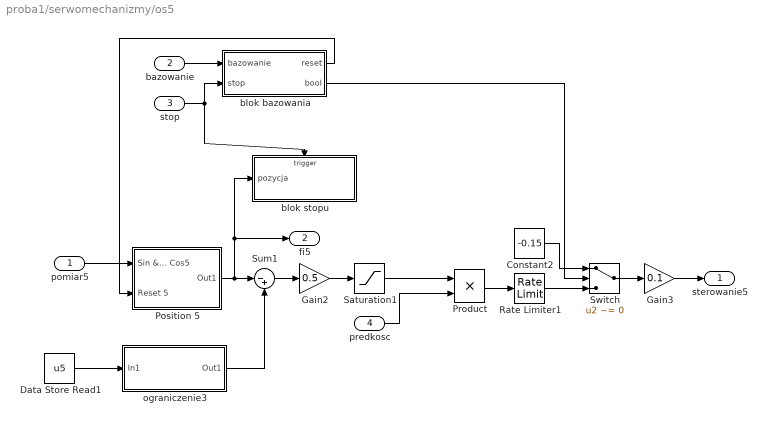
== system proba1/serwomechanizmy/os5 ==
  pomiar5 : Inport
  bazowanie : Inport  Port=2
  stop : Inport  Port=3
  predkosc : Inport  Port=4
  Constant2 : Constant  Value=-0.15
  Data Store Read1 : DataStoreRead  DataStoreName=u5  SampleTime=0
  Gain2 : Gain  Gain=0.5
  Gain3 : Gain  Gain=0.1
  Position 5 : Subsystem
  Product : Product  RndMeth=Zero
  Rate Limiter1 : RateLimiter  RisingSlewLimit=50  FallingSlewLimit=-50  SampleTimeMode=inherited
  Saturation1 : Saturate  UpperLimit=3  LowerLimit=-3
  Sum1 : Sum  Inputs=|-+
  Switch : Switch  Criteria=u2 ~= 0
  blok bazowania : Subsystem
  blok stopu : Subsystem  TreatAsAtomicUnit=on
  ograniczenie3 : Subsystem
  sterowanie5 : Outport
  fi5 : Outport  Port=2
  wires:
  Sum1/1 -> Gain2/1
  pomiar5/1 -> Position 5/1(Sin && Cos5)
  Position 5/1(Out1) -> Sum1/1, fi5/1, blok stopu/1(pozycja)
  Gain3/1 -> sterowanie5/1
  Data Store Read1/1 -> ograniczenie3/1(In1)
  ograniczenie3/1(Out1) -> Sum1/2
  Gain2/1 -> Saturation1/1
  Saturation1/1 -> Product/1
  predkosc/1 -> Product/2
  Product/1 -> Rate Limiter1/1
  Constant2/1 -> Switch/1
  Switch/1 -> Gain3/1
  Rate Limiter1/1 -> Switch/3
  blok bazowania/2(bool) -> Switch/2
  blok bazowania/1(reset) -> Position 5/2(Reset 5)
  bazowanie/1 -> blok bazowania/1(bazowanie)
  stop/1 -> blok stopu/Trigger, blok bazowania/2(stop)

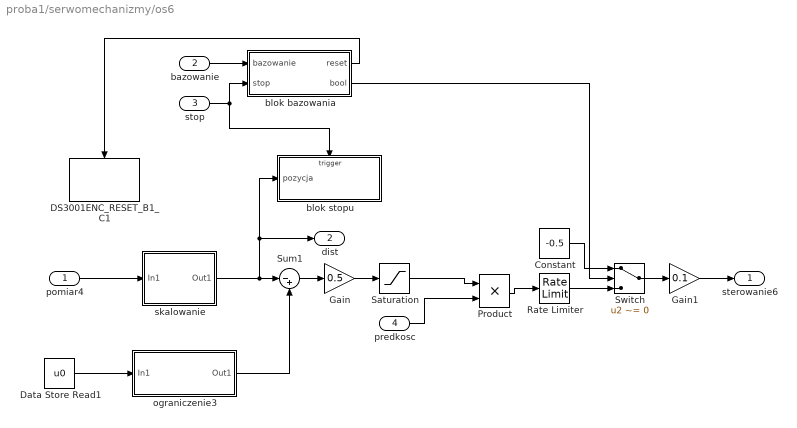
== system proba1/serwomechanizmy/os6 ==
  pomiar4 : Inport
  bazowanie : Inport  Port=2
  stop : Inport  Port=3
  predkosc : Inport  Port=4
  Constant : Constant  Value=-0.5
  DS3001ENC_RESET_B1_C1 : rtilibm/DS3001/DS3001ENC_RESET_B1_C1  SystemSampleTime=-1  BoardNo=1  ChannelNo=1  DialogFcn=gui3001enc_reset_c  UnitName={ 'DS3001ENC_RESET_B', '_C' }  UnitValues="{1  1}"  DSProperties=struct('RTI',struct('Version',uint32(1),'BlockType',struct('isSLSource',uint8(0),'isSLSink',uint8(1),'isHWSource',uint8(0),'isHWSink',uint8(1),'isSetup',uint8(0),'isInline',uint8(1),'isNonInline',uint8(0),'isInterrupt',uint8(0),'isChannelwise',uint8(1)),'IOBoardType','DS3001','UnitType','ENC','Identifier','ENCRESET','DialogType','ML','BlockSet','NONE','SlaveProcessor','NONE'))
  Data Store Read1 : DataStoreRead  DataStoreName=u0  SampleTime=0
  Gain : Gain  Gain=0.5
  Gain1 : Gain  Gain=0.1
  Product : Product  RndMeth=Zero
  Rate Limiter : RateLimiter  RisingSlewLimit=50  FallingSlewLimit=-50  SampleTimeMode=inherited
  Saturation : Saturate  UpperLimit=3  LowerLimit=-3
  Sum1 : Sum  Inputs=|-+
  Switch : Switch  Criteria=u2 ~= 0
  blok bazowania : Subsystem
  blok stopu : Subsystem  TreatAsAtomicUnit=on
  ograniczenie3 : Subsystem
  skalowanie : Subsystem
  sterowanie6 : Outport
  dist : Outport  Port=2
  wires:
  Sum1/1 -> Gain/1
  skalowanie/1(Out1) -> Sum1/1, dist/1, blok stopu/1(pozycja)
  Gain1/1 -> sterowanie6/1
  Data Store Read1/1 -> ograniczenie3/1(In1)
  ograniczenie3/1(Out1) -> Sum1/2
  Gain/1 -> Saturation/1
  Saturation/1 -> Product/1
  predkosc/1 -> Product/2
  Product/1 -> Rate Limiter/1
  Constant/1 -> Switch/1
  Switch/1 -> Gain1/1
  Rate Limiter/1 -> Switch/3
  blok bazowania/2(bool) -> Switch/2
  blok bazowania/1(reset) -> DS3001ENC_RESET_B1_C1/Trigger
  bazowanie/1 -> blok bazowania/1(bazowanie)
  stop/1 -> blok bazowania/2(stop), blok stopu/Trigger
  pomiar4/1 -> skalowanie/1(In1)

== system proba1/serwomechanizmy/quasiliniowosc ==
  E3 : Inport
  E2 : Inport  Port=2
  E1 : Inport  Port=3
  Abs : Abs
  Abs1 : Abs
  Abs2 : Abs
  Divide : Product  Inputs=*/
  Divide1 : Product  Inputs=*/
  Divide2 : Product  Inputs=*/
  MinMax : MinMax  Function=max  Inputs=3
  Saturation : Saturate  UpperLimit=1  LowerLimit=0.05
  Saturation1 : Saturate  UpperLimit=1  LowerLimit=0.05
  Saturation2 : Saturate  UpperLimit=1  LowerLimit=0.05
  wspE3 : Outport
  wspE2 : Outport  Port=2
  wspE1 : Outport  Port=3
  wires:
  E1/1 -> Abs/1
  E2/1 -> Abs1/1
  E3/1 -> Abs2/1
  Abs1/1 -> MinMax/2, Divide1/1
  Divide/1 -> Saturation/1
  Abs2/1 -> MinMax/3, Divide2/1
  Abs/1 -> Divide/1, MinMax/1
  Divide1/1 -> Saturation1/1
  Divide2/1 -> Saturation2/1
  MinMax/1 -> Divide/2, Divide1/2, Divide2/2
  Saturation/1 -> wspE1/1
  Saturation1/1 -> wspE2/1
  Saturation2/1 -> wspE3/1

== system proba1/tryby/jedz do przedmiotu ==
  Enable : EnablePort
  Trigger : TriggerPort
  Data Store Read : DataStoreRead  DataStoreName=obliczoneFi1  SampleTime=-1
  Data Store Read1 : DataStoreRead  DataStoreName=obliczoneFi3  SampleTime=-1
  Data Store Read2 : DataStoreRead  DataStoreName=obliczoneFi2  SampleTime=-1
  Data Store Read3 : DataStoreRead  DataStoreName=obliczoneDist  SampleTime=-1
  Data Store Write : DataStoreWrite  DataStoreName=tmp_u1  SampleTime=-1
  Data Store Write1 : DataStoreWrite  DataStoreName=tmp_u2  SampleTime=-1
  Data Store Write2 : DataStoreWrite  DataStoreName=tmp_u3  SampleTime=-1
  Data Store Write3 : DataStoreWrite  DataStoreName=u1  SampleTime=-1
  Data Store Write4 : DataStoreWrite  DataStoreName=u2  SampleTime=-1
  Data Store Write5 : DataStoreWrite  DataStoreName=u3  SampleTime=-1
  Data Store Write6 : DataStoreWrite  DataStoreName=tmp_u0  SampleTime=-1
  Data Store Write7 : DataStoreWrite  DataStoreName=u0  SampleTime=-1
  wires:
  Data Store Read/1 -> Data Store Write/1, Data Store Write3/1
  Data Store Read2/1 -> Data Store Write1/1, Data Store Write4/1
  Data Store Read1/1 -> Data Store Write2/1, Data Store Write5/1
  Data Store Read3/1 -> Data Store Write6/1, Data Store Write7/1

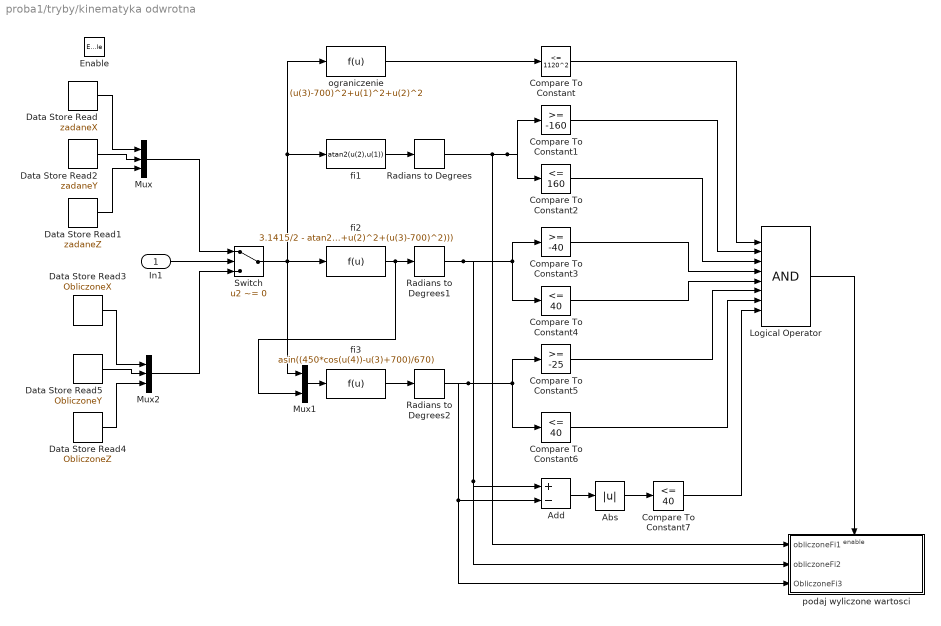
== system proba1/tryby/kinematyka odwrotna ==
  In1 : Inport  OutDataType=sfix(16)  OutScaling=2^0
  Enable : EnablePort
  Abs : Abs
  Add : Sum  Inputs=+-
  Compare To Constant : simulink/Logic and Bit Operations/Compare To Constant  SystemSampleTime=-1  relop=<=  const=1120^2  LogicOutDataTypeMode=boolean  ZeroCross=off
  Compare To Constant1 : simulink/Logic and Bit Operations/Compare To Constant  SystemSampleTime=-1  relop=>=  const=-160  LogicOutDataTypeMode=boolean  ZeroCross=off
  Compare To Constant2 : simulink/Logic and Bit Operations/Compare To Constant  SystemSampleTime=-1  relop=<=  const=160  LogicOutDataTypeMode=boolean  ZeroCross=off
  Compare To Constant3 : simulink/Logic and Bit Operations/Compare To Constant  SystemSampleTime=-1  relop=>=  const=-40  LogicOutDataTypeMode=boolean  ZeroCross=off
  Compare To Constant4 : simulink/Logic and Bit Operations/Compare To Constant  SystemSampleTime=-1  relop=<=  const=40  LogicOutDataTypeMode=boolean  ZeroCross=off
  Compare To Constant5 : simulink/Logic and Bit Operations/Compare To Constant  SystemSampleTime=-1  relop=>=  const=-25  LogicOutDataTypeMode=boolean  ZeroCross=off
  Compare To Constant6 : simulink/Logic and Bit Operations/Compare To Constant  SystemSampleTime=-1  relop=<=  const=40  LogicOutDataTypeMode=boolean  ZeroCross=off
  Compare To Constant7 : simulink/Logic and Bit Operations/Compare To Constant  SystemSampleTime=-1  relop=<=  const=40  LogicOutDataTypeMode=boolean  ZeroCross=off
  Data Store Read : DataStoreRead  DataStoreName=zadaneX  SampleTime=0
  Data Store Read1 : DataStoreRead  DataStoreName=zadaneZ  SampleTime=0
  Data Store Read2 : DataStoreRead  DataStoreName=zadaneY  SampleTime=0
  Data Store Read3 : DataStoreRead  DataStoreName=ObliczoneX  SampleTime=0
  Data Store Read4 : DataStoreRead  DataStoreName=ObliczoneZ  SampleTime=0
  Data Store Read5 : DataStoreRead  DataStoreName=ObliczoneY  SampleTime=0
  Logical Operator : Logic  Inputs=8  AllPortsSameDT=off  OutDataTypeMode=boolean
  Mux : Mux  Inputs=3
  Mux1 : Mux  Inputs=2
  Mux2 : Mux  Inputs=3
  Radians to Degrees : simulink_extras/Transformations/Radians to Degrees  SystemSampleTime=-1
  Radians to Degrees1 : simulink_extras/Transformations/Radians to Degrees  SystemSampleTime=-1
  Radians to Degrees2 : simulink_extras/Transformations/Radians to Degrees  SystemSampleTime=-1
  Switch : Switch  Criteria=u2 ~= 0  OutDataType=sfix(16)  OutScaling=2^0
  fi1 : Fcn  Expr=atan2(u(2),u(1))
  fi2 : Fcn  Expr=3.1415/2 - atan2((u(3)-700),sqrt(u(1)^2+u(2)^2)) - acos((450^2+u(1)^2+u(2)^2+(u(3)-700)^2-670^2)/(2*450*sqrt(u(1)^2+u(2)^2+(u(3)-700)^2)))
  fi3 : Fcn  Expr=asin((450*cos(u(4))-u(3)+700)/670)
  ograniczenie : Fcn  Expr=(u(3)-700)^2+u(1)^2+u(2)^2
  podaj wyliczone wartosci : Subsystem  TreatAsAtomicUnit=on
  wires:
  fi1/1 -> Radians to Degrees/1
  ograniczenie/1 -> Compare To Constant/1
  Radians to Degrees/1 -> Compare To Constant1/1, Compare To Constant2/1, podaj wyliczone wartosci/1(obliczoneFi1)
  Add/1 -> Abs/1
  Abs/1 -> Compare To Constant7/1
  Radians to Degrees1/1 -> Compare To Constant3/1, Compare To Constant4/1, Add/1, podaj wyliczone wartosci/2(obliczoneFi2)
  fi3/1 -> Radians to Degrees2/1
  fi2/1 -> Radians to Degrees1/1, Mux1/2
  Radians to Degrees2/1 -> Compare To Constant5/1, Compare To Constant6/1, Add/2, podaj wyliczone wartosci/3(ObliczoneFi3)
  Compare To Constant7/1 -> Logical Operator/8
  Compare To Constant/1 -> Logical Operator/1
  Compare To Constant1/1 -> Logical Operator/2
  Compare To Constant2/1 -> Logical Operator/3
  Compare To Constant3/1 -> Logical Operator/4
  Compare To Constant4/1 -> Logical Operator/5
  Compare To Constant5/1 -> Logical Operator/6
  Compare To Constant6/1 -> Logical Operator/7
  Logical Operator/1 -> podaj wyliczone wartosci/Enable
  Mux1/1 -> fi3/1
  Switch/1 -> ograniczenie/1, fi1/1, fi2/1, Mux1/1
  In1/1 -> Switch/2
  Data Store Read3/1 -> Mux2/1
  Data Store Read5/1 -> Mux2/2
  Data Store Read4/1 -> Mux2/3
  Mux2/1 -> Switch/3
  Data Store Read/1 -> Mux/1
  Data Store Read2/1 -> Mux/2
  Data Store Read1/1 -> Mux/3
  Mux/1 -> Switch/1

== system proba1/tryby/rozpoznawanie obrazu ==
  Enable : EnablePort
  Trigger : TriggerPort
  Constant : Constant  Value=212  OutDataType=sfix(16)  OutScaling=2^0
  Constant1 : Constant  Value=0  OutDataType=sfix(16)  OutScaling=2^0
  Data Store Write : DataStoreWrite  DataStoreName=zadaneX  SampleTime=-1
  Data Store Write1 : DataStoreWrite  DataStoreName=zadaneY  SampleTime=-1
  Data Store Write2 : DataStoreWrite  DataStoreName=zadaneZ  SampleTime=-1
  Data Store Write3 : DataStoreWrite  DataStoreName=A  SampleTime=-1
  Detect Change : simulink/Logic and Bit Operations/Detect Change  SystemSampleTime=-1  vinit=0
  Detect Change1 : simulink/Logic and Bit Operations/Detect Change  SystemSampleTime=-1  vinit=0
  Detect Change2 : simulink/Logic and Bit Operations/Detect Change  SystemSampleTime=-1  vinit=0
  Embedded MATLAB Function : Stateflow chart
  Logical Operator : Logic  Inputs=3  AllPortsSameDT=off  OutDataTypeMode=boolean
  Scope : Scope  NumInputPorts=3
      settings: YMin=-5~-5~-5  YMax=5~5~5
  podaj wyliczone wartosci : Subsystem  TreatAsAtomicUnit=on
  gotowy : Outport  OutDataType=sfix(16)  OutScaling=2^0
  wires:
  Embedded MATLAB Function/1(x) -> podaj wyliczone wartosci/1(zadaneX), Detect Change/1, Scope/1, Data Store Write/1
  Embedded MATLAB Function/2(y) -> podaj wyliczone wartosci/2(zadaneY), Detect Change1/1, Scope/2, Data Store Write1/1
  Embedded MATLAB Function/3(z) -> podaj wyliczone wartosci/3(zadaneZ), Detect Change2/1, Scope/3, Data Store Write2/1
  Detect Change/1 -> Logical Operator/1
  Detect Change1/1 -> Logical Operator/2
  Detect Change2/1 -> Logical Operator/3
  Logical Operator/1 -> gotowy/1
  Constant/1 -> Data Store Write3/1
  Constant1/1 -> Embedded MATLAB Function/1(k)

== system proba1/tryby/tryb ciagly ==
  Enable : EnablePort
  Data Store Read : DataStoreRead  DataStoreName=tmp_u2  SampleTime=-1
  Data Store Read1 : DataStoreRead  DataStoreName=tmp_u3  SampleTime=-1
  Data Store Read2 : DataStoreRead  DataStoreName=tmp_u1  SampleTime=-1
  Data Store Read3 : DataStoreRead  DataStoreName=tmp_u0  SampleTime=-1
  Data Store Read4 : DataStoreRead  DataStoreName=tmp_u4  SampleTime=-1
  Data Store Read5 : DataStoreRead  DataStoreName=tmp_u5  SampleTime=-1
  Data Store Write : DataStoreWrite  DataStoreName=u1  SampleTime=-1
  Data Store Write1 : DataStoreWrite  DataStoreName=u2  SampleTime=-1
  Data Store Write2 : DataStoreWrite  DataStoreName=u3  SampleTime=-1
  Data Store Write3 : DataStoreWrite  DataStoreName=u0  SampleTime=-1
  Data Store Write4 : DataStoreWrite  DataStoreName=u4  SampleTime=-1
  Data Store Write5 : DataStoreWrite  DataStoreName=u5  SampleTime=-1
  wires:
  Data Store Read2/1 -> Data Store Write/1
  Data Store Read/1 -> Data Store Write1/1
  Data Store Read1/1 -> Data Store Write2/1
  Data Store Read3/1 -> Data Store Write3/1
  Data Store Read4/1 -> Data Store Write4/1
  Data Store Read5/1 -> Data Store Write5/1

== system proba1/tryby/tryb kinematyki odwrotnej ==
  Enable : EnablePort
  Trigger : TriggerPort
  Data Store Read : DataStoreRead  DataStoreName=obliczoneFi1  SampleTime=-1
  Data Store Read1 : DataStoreRead  DataStoreName=obliczoneFi3  SampleTime=-1
  Data Store Read2 : DataStoreRead  DataStoreName=obliczoneFi2  SampleTime=-1
  Data Store Read3 : DataStoreRead  DataStoreName=obliczoneDist  SampleTime=-1
  Data Store Write : DataStoreWrite  DataStoreName=tmp_u1  SampleTime=-1
  Data Store Write1 : DataStoreWrite  DataStoreName=tmp_u2  SampleTime=-1
  Data Store Write2 : DataStoreWrite  DataStoreName=tmp_u3  SampleTime=-1
  Data Store Write3 : DataStoreWrite  DataStoreName=u1  SampleTime=-1
  Data Store Write4 : DataStoreWrite  DataStoreName=u2  SampleTime=-1
  Data Store Write5 : DataStoreWrite  DataStoreName=u3  SampleTime=-1
  Data Store Write6 : DataStoreWrite  DataStoreName=tmp_u0  SampleTime=-1
  Data Store Write7 : DataStoreWrite  DataStoreName=u0  SampleTime=-1
  wires:
  Data Store Read/1 -> Data Store Write/1, Data Store Write3/1
  Data Store Read2/1 -> Data Store Write1/1, Data Store Write4/1
  Data Store Read1/1 -> Data Store Write2/1, Data Store Write5/1
  Data Store Read3/1 -> Data Store Write6/1, Data Store Write7/1

== system proba1/tryby/tryb wyzwalany ==
  Enable : EnablePort
  Trigger : TriggerPort
  Data Store Read : DataStoreRead  DataStoreName=tmp_u2  SampleTime=-1
  Data Store Read1 : DataStoreRead  DataStoreName=tmp_u3  SampleTime=-1
  Data Store Read2 : DataStoreRead  DataStoreName=tmp_u1  SampleTime=-1
  Data Store Read3 : DataStoreRead  DataStoreName=tmp_u4  SampleTime=-1
  Data Store Read4 : DataStoreRead  DataStoreName=tmp_u0  SampleTime=-1
  Data Store Read5 : DataStoreRead  DataStoreName=tmp_u5  SampleTime=-1
  Data Store Write : DataStoreWrite  DataStoreName=u1  SampleTime=-1
  Data Store Write1 : DataStoreWrite  DataStoreName=u2  SampleTime=-1
  Data Store Write2 : DataStoreWrite  DataStoreName=u3  SampleTime=-1
  Data Store Write3 : DataStoreWrite  DataStoreName=u4  SampleTime=-1
  Data Store Write4 : DataStoreWrite  DataStoreName=u0  SampleTime=-1
  Data Store Write5 : DataStoreWrite  DataStoreName=u5  SampleTime=-1
  wires:
  Data Store Read2/1 -> Data Store Write/1
  Data Store Read/1 -> Data Store Write1/1
  Data Store Read1/1 -> Data Store Write2/1
  Data Store Read3/1 -> Data Store Write3/1
  Data Store Read4/1 -> Data Store Write4/1
  Data Store Read5/1 -> Data Store Write5/1

== system proba1/RTI Data/RTI Data Store/RTI Data Store ==
  RTI Data Store : Subsystem
      mask Type: RTI_DATA_STORE
      mask Description:
      | RTI Data Store Block. This block is used by RTI to store internal model dependent data. Deleting this block will result in data loss.
      | 
      | NEVER DELETE, COPY, OR MODIFY THIS BLOCK!
      mask Help:
      | RTI Data Store Block. This block is used by RTI to store internal model dependent data. Deleting this block will result in data loss.
      | 
      | NEVER DELETE, COPY, OR MODIFY THIS BLOCK!
      mask Display: text(0.5, 0.5, ' ', 'HorizontalAlignment', 'center');

== system proba1/serwomechanizmy/os1/Position 1 ==
  Sin && Cos1 : Inport
  Reset 1 : Inport  Port=2
  Filters 1 : Subsystem
  Position Calculation 1 : Subsystem
  Out1 : Outport
  wires:
  Filters 1/1(Sin) -> Position Calculation 1/1(Sin)
  Filters 1/2(Cos) -> Position Calculation 1/2(Cos)
  Sin && Cos1/1 -> Filters 1/1(Sin && Cos)
  Reset 1/1 -> Position Calculation 1/3(Reset (Impulse))
  Position Calculation 1/1(Position) -> Out1/1

== system proba1/serwomechanizmy/os1/blok bazowania ==
  bazowanie : Inport
  stop : Inport  Port=2
  DS2201IN_B1 : rtilibm/DS2201/DS2201IN_B1  SystemSampleTime=-1  BoardNo=1  ChannelNos=1  DialogFcn=gui2201in  UnitName={ 'DS2201IN_B' }  UnitValues={ 1 }  DSProperties=struct('RTI',struct('Version',uint32(1),'BlockType',struct('isSLSource',uint8(1),'isSLSink',uint8(0),'isHWSource',uint8(1),'isHWSink',uint8(0),'isSetup',uint8(0),'isInline',uint8(1),'isNonInline',uint8(0),'isInterrupt',uint8(0),'isChannelwise',uint8(0)),'IOBoardType','DS2201','UnitType','BIT','Identifier','BITIN','DialogType','ML','BlockSet','NONE','SlaveProcessor','NONE'))
  Logical Operator : Logic  Operator=OR  AllPortsSameDT=off
  S-R Flip-Flop : simulink_extras/Flip Flops/S-R Flip-Flop  SystemSampleTime=-1  initial_condition=0
  zerowanie : Subsystem  TreatAsAtomicUnit=on
  reset : Outport
  bool : Outport  Port=2
  wires:
  bazowanie/1 -> S-R Flip-Flop/1
  S-R Flip-Flop/1 -> bool/1, zerowanie/Enable
  S-R Flip-Flop/2 -> reset/1
  DS2201IN_B1/1 -> Logical Operator/1
  stop/1 -> Logical Operator/2
  Logical Operator/1 -> S-R Flip-Flop/2

== system proba1/serwomechanizmy/os1/blok stopu ==
  pozycja : Inport
  Trigger : TriggerPort
  Data Store Write : DataStoreWrite  DataStoreName=u1  SampleTime=-1
  Data Store Write1 : DataStoreWrite  DataStoreName=tmp_u1  SampleTime=-1
  wires:
  pozycja/1 -> Data Store Write/1, Data Store Write1/1

== system proba1/serwomechanizmy/os1/ograniczenie1 ==
  In1 : Inport
  Compare To Constant : simulink/Logic and Bit Operations/Compare To Constant  SystemSampleTime=-1  relop=<=  const=160  LogicOutDataTypeMode=boolean  ZeroCross=off
  Compare To Constant1 : simulink/Logic and Bit Operations/Compare To Constant  SystemSampleTime=-1  relop=>=  const=-160  LogicOutDataTypeMode=boolean  ZeroCross=off
  Constant1 : Constant  Value=0
  Logical Operator : Logic  AllPortsSameDT=off  OutDataTypeMode=boolean
  Switch : Switch  Criteria=u2 ~= 0
  Out1 : Outport
  wires:
  In1/1 -> Compare To Constant/1, Compare To Constant1/1, Switch/1
  Compare To Constant1/1 -> Logical Operator/1
  Compare To Constant/1 -> Logical Operator/2
  Logical Operator/1 -> Switch/2
  Constant1/1 -> Switch/3
  Switch/1 -> Out1/1

== system proba1/serwomechanizmy/os2/Position 2 ==
  Sin && Cos2 : Inport
  Reset 2 : Inport  Port=2
  Filters 2 : Subsystem
  Position Calculation 2 : Subsystem
  Out1 : Outport
  wires:
  Filters 2/1(Sin) -> Position Calculation 2/1(Sin)
  Filters 2/2(Cos) -> Position Calculation 2/2(Cos)
  Sin && Cos2/1 -> Filters 2/1(Sin && Cos)
  Reset 2/1 -> Position Calculation 2/3(Reset (Impulse))
  Position Calculation 2/1(Position) -> Out1/1

== system proba1/serwomechanizmy/os2/blok bazowania ==
  bazowanie : Inport
  stop : Inport  Port=2
  DS2201IN_B1 : rtilibm/DS2201/DS2201IN_B1  SystemSampleTime=-1  BoardNo=1  ChannelNos=2  DialogFcn=gui2201in  UnitName={ 'DS2201IN_B' }  UnitValues={ 1 }  DSProperties=struct('RTI',struct('Version',uint32(1),'BlockType',struct('isSLSource',uint8(1),'isSLSink',uint8(0),'isHWSource',uint8(1),'isHWSink',uint8(0),'isSetup',uint8(0),'isInline',uint8(1),'isNonInline',uint8(0),'isInterrupt',uint8(0),'isChannelwise',uint8(0)),'IOBoardType','DS2201','UnitType','BIT','Identifier','BITIN','DialogType','ML','BlockSet','NONE','SlaveProcessor','NONE'))
  Logical Operator : Logic  Operator=OR  AllPortsSameDT=off
  S-R Flip-Flop : simulink_extras/Flip Flops/S-R Flip-Flop  SystemSampleTime=-1  initial_condition=0
  zerowanie : Subsystem  TreatAsAtomicUnit=on
  reset : Outport
  bool : Outport  Port=2
  wires:
  bazowanie/1 -> S-R Flip-Flop/1
  S-R Flip-Flop/1 -> bool/1, zerowanie/Enable
  S-R Flip-Flop/2 -> reset/1
  stop/1 -> Logical Operator/2
  Logical Operator/1 -> S-R Flip-Flop/2
  DS2201IN_B1/1 -> Logical Operator/1

== system proba1/serwomechanizmy/os2/blok stopu ==
  pozycja : Inport
  Trigger : TriggerPort
  Data Store Write : DataStoreWrite  DataStoreName=u2  SampleTime=-1
  Data Store Write1 : DataStoreWrite  DataStoreName=tmp_u2  SampleTime=-1
  wires:
  pozycja/1 -> Data Store Write/1, Data Store Write1/1

== system proba1/serwomechanizmy/os2/ograniczenie2 ==
  In1 : Inport
  Compare To Constant : simulink/Logic and Bit Operations/Compare To Constant  SystemSampleTime=-1  relop=<=  const=40  LogicOutDataTypeMode=boolean  ZeroCross=off
  Compare To Constant1 : simulink/Logic and Bit Operations/Compare To Constant  SystemSampleTime=-1  relop=>=  const=-40  LogicOutDataTypeMode=boolean  ZeroCross=off
  Constant1 : Constant  Value=0
  Logical Operator : Logic  AllPortsSameDT=off  OutDataTypeMode=boolean
  Switch : Switch  Criteria=u2 ~= 0
  Out1 : Outport
  wires:
  In1/1 -> Compare To Constant/1, Compare To Constant1/1, Switch/1
  Compare To Constant1/1 -> Logical Operator/1
  Compare To Constant/1 -> Logical Operator/2
  Logical Operator/1 -> Switch/2
  Constant1/1 -> Switch/3
  Switch/1 -> Out1/1

== system proba1/serwomechanizmy/os3/Position 3 ==
  Sin && Cos3 : Inport
  Reset 3 : Inport  Port=2
  Filters 3 : Subsystem
  Position Calculation 3 : Subsystem
  Out1 : Outport
  wires:
  Filters 3/1(Sin) -> Position Calculation 3/1(Sin)
  Filters 3/2(Cos) -> Position Calculation 3/2(Cos)
  Sin && Cos3/1 -> Filters 3/1(Sin && Cos)
  Reset 3/1 -> Position Calculation 3/3(Reset (Impulse))
  Position Calculation 3/1(Position) -> Out1/1

== system proba1/serwomechanizmy/os3/blok bazowania ==
  bazowanie : Inport
  stop : Inport  Port=2
  DS2201IN_B1 : rtilibm/DS2201/DS2201IN_B1  SystemSampleTime=-1  BoardNo=1  ChannelNos=3  DialogFcn=gui2201in  UnitName={ 'DS2201IN_B' }  UnitValues={ 1 }  DSProperties=struct('RTI',struct('Version',uint32(1),'BlockType',struct('isSLSource',uint8(1),'isSLSink',uint8(0),'isHWSource',uint8(1),'isHWSink',uint8(0),'isSetup',uint8(0),'isInline',uint8(1),'isNonInline',uint8(0),'isInterrupt',uint8(0),'isChannelwise',uint8(0)),'IOBoardType','DS2201','UnitType','BIT','Identifier','BITIN','DialogType','ML','BlockSet','NONE','SlaveProcessor','NONE'))
  Logical Operator : Logic  Operator=OR  AllPortsSameDT=off
  S-R Flip-Flop : simulink_extras/Flip Flops/S-R Flip-Flop  SystemSampleTime=-1  initial_condition=0
  zerowanie : Subsystem  TreatAsAtomicUnit=on
  reset : Outport
  bool : Outport  Port=2
  wires:
  bazowanie/1 -> S-R Flip-Flop/1
  S-R Flip-Flop/1 -> bool/1, zerowanie/Enable
  S-R Flip-Flop/2 -> reset/1
  stop/1 -> Logical Operator/2
  DS2201IN_B1/1 -> Logical Operator/1
  Logical Operator/1 -> S-R Flip-Flop/2

== system proba1/serwomechanizmy/os3/blok stopu ==
  pozycja : Inport
  Trigger : TriggerPort
  Data Store Write : DataStoreWrite  DataStoreName=u3  SampleTime=-1
  Data Store Write1 : DataStoreWrite  DataStoreName=tmp_u3  SampleTime=-1
  wires:
  pozycja/1 -> Data Store Write/1, Data Store Write1/1
